simulink model "KD_cl_harness_forthao_breach"  (R2015a)
settings: Solver=ode45  StartTime=0  StopTime=50  FixedStep=0.01  MaxStep=0.005  RelTol=1e-4  AbsTol=1e-4
InitFcn:
  | load KD_const_coeffs_0624
  | load pexhat_stuff
  | load expcon
  | load thr_ff_map
undefined symbols (not defined in the file): c_0, c_1, c_100, c_1000, c_10000, c_1000inv, c_100inv, c_1_int, c_1d2p4, c_1p7, c_4400inv, c_5500inv, c_80, c_90, c_cal_phi, c_compmap, c_ctok, c_fflow_max, c_fflow_min, c_filt, c_flowdiv, c_flowmin, c_flowmult, c_inf, c_km1d2k, c_mm3tokgpers, c_n1, c_p00001, c_p01, c_p016, c_p1429, c_p1e9, c_p4167, c_p4d1p4, c_p5401, c_p9, c_pincomp, c_ra, c_rair, c_Rby1000, c_roacorr, c_rpmtoradpers, c_svrthrottle1, c_svrthrottle2, c_svrthrottlearg, c_svrthrottlebeta, c_ta_max, c_ta_min, c_V, c_vnliftmax, c_vnliftmin, Coefs, const, const_exhat, eegr_map, egrr_delay_init, epim_map, eplufin_ff_map, expcon, invta ... (+17)
libraries: simulink x5
(part 5 of 5)

== system KD_cl_harness_forthao_breach/ctrl_rb_explicit_20131031_v2/While_Iterator_Subsystem/newton/update ==
  dwdp : Inport
  error : Inport  Port=2
  Data Store Read1 : DataStoreRead  DataStoreName=man_pex_eps
  Data Store Read11 : DataStoreRead  DataStoreName=man_pex_eps
  Data Store Read16 : DataStoreRead  DataStoreName=man_use_LM
  Product2 : Product  Inputs=**  RndMeth=Zero
  Product3 : Product  Inputs=/*  RndMeth=Zero
  Product8 : Product  Inputs=/**  RndMeth=Zero
  Relational Operator7 : RelationalOperator  Operator=>  OutDataTypeStr=boolean
      settings: AttributesFormatString=%<Operator>
  Saturation1 : Saturate  UpperLimit=c_inf  LowerLimit=c_p1e9
      settings: AttributesFormatString=%<LowerLimit>\n%<UpperLimit>
  Saturation3 : Saturate  UpperLimit=c_inf  LowerLimit=c_p1e9
      settings: AttributesFormatString=%<LowerLimit>\n%<UpperLimit>
  Sum1 : Sum  Inputs=|++
  Sum2 : Sum  Inputs=|++
  Switch7 : Switch  Criteria=u2 ~= 0
      settings: AttributesFormatString=%<Criteria>
  man_pex_eps : Gain
  man_pex_eps1 : Gain
  man_use_LM : Gain
  zero8 : Constant  Value=0  OutDataTypeStr=single  SampleTime=-1
      settings: AttributesFormatString=%<Value>\n%<SampleTime>
  delta : Outport
  wires:
  Data Store Read11/1 -> man_pex_eps/1
  Sum2/1 -> Saturation3/1
  Saturation3/1 -> Product8/1
  Product2/1 -> Sum2/2
  error/1 -> [e]
  dwdp/1 -> [dwdp]
  [dwdp] -> Product2/1, Product8/2, Product2/2
  [e] -> Product8/3
  Data Store Read1/1 -> man_pex_eps1/1
  Sum1/1 -> Saturation1/1
  Saturation1/1 -> Product3/1
  [dwdp] -> Sum1/2
  [e] -> Product3/2
  zero8/1 -> Relational Operator7/2
  Data Store Read16/1 -> man_use_LM/1
  Relational Operator7/1 -> Switch7/2
  Product3/1 -> Switch7/3
  Product8/1 -> Switch7/1
  Switch7/1 -> delta/1
  man_pex_eps/1 -> Sum2/1
  man_pex_eps1/1 -> Sum1/1
  man_use_LM/1 -> Relational Operator7/1

== system KD_cl_harness_forthao_breach/ctrl_rb_explicit_20131031_v2/expcon/find_region/find_region ==
  u : Inport
  IC : Inport  Port=2
  Constant : Constant  DisableCoverage=on  Value=c_0  OutDataTypeStr=Inherit: Inherit via back propagation  PreserveConstantTs=on
      settings: AttributesFormatString=%<Value>
  g_zero_continue : RelationalOperator  Operator=>  OutDataTypeStr=boolean  InputSameDT=on
  get_region_violation : Subsystem
  if_region_1 : SwitchCase
  leq_check : Subsystem
  reg_register : UnitDelay  InitialCondition=c_1_int  SampleTime=-1
      settings: AttributesFormatString=%<X0>
  reg_update_merge : Merge  Inputs=3  InitialOutput=c_1_int
      settings: AttributesFormatString=%<InitialOutput>
  region_1feedthrough : Subsystem  TreatAsAtomicUnit=on
  region_iter : WhileIterator  MaxIters=expcon.Nr  ShowIterationPort=on
  rv_register : UnitDelay  InitialCondition=c_10000  SampleTime=-1
      settings: AttributesFormatString=%<X0>
  rv_update_merge : Merge  Inputs=3  InitialOutput=c_10000
      settings: AttributesFormatString=%<InitialOutput>
  region : Outport  InitialOutput=c_1_int
      settings: AttributesFormatString=%<InitialOutput>
  rv : Outport  Port=2  InitialOutput=c_10000
      settings: AttributesFormatString=%<InitialOutput>
  wires:
  region_iter/1 -> [iter]
  [iter] -> if_region_1/1, get_region_violation/1(region), leq_check/2(region_ind)
  IC/1 -> region_iter/2
  Constant/1 -> g_zero_continue/2
  [reg] -> reg_update_merge/1
  region_1feedthrough/2(region) -> [reg]
  [def] -> leq_check/Action
  if_region_1/2 -> [def]
  [u] -> get_region_violation/2(u)
  u/1 -> [u]
  get_region_violation/1(region_violation) -> region_1feedthrough/1(rvin), leq_check/1(rv_new)
  leq_check/1(rv_update_new) -> rv_update_merge/2
  rv_register/1 -> leq_check/3(rv_old)
  g_zero_continue/1 -> region_iter/1
  leq_check/3(region_update_new) -> reg_update_merge/2
  reg_register/1 -> leq_check/4(region_old)
  reg_update_merge/1 -> reg_register/1, region/1
  rv_update_merge/1 -> g_zero_continue/1, rv_register/1, rv/1
  region_1feedthrough/1(rvout) -> rv_update_merge/1
  if_region_1/1 -> region_1feedthrough/Action
  leq_check/2(rv_update_old) -> rv_update_merge/3
  leq_check/4(region_updateold) -> reg_update_merge/3

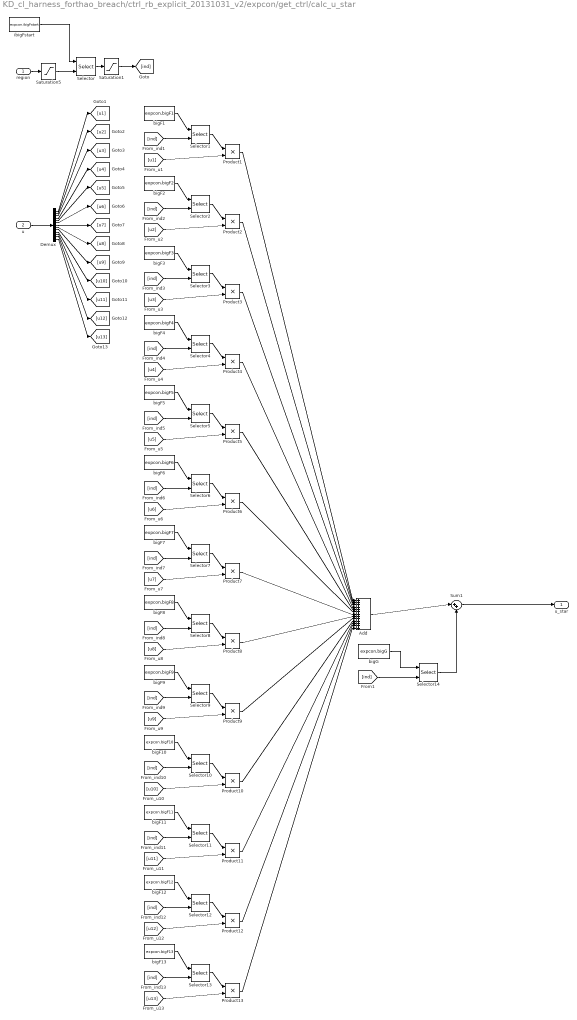
== system KD_cl_harness_forthao_breach/ctrl_rb_explicit_20131031_v2/expcon/get_ctrl/calc_u_star ==
  region : Inport
  u : Inport  Port=2
  Add : Sum  Inputs=+++++++++++++
  Demux : Demux  Outputs=13
  Product{1..13} (13 alike) : Product  RndMeth=Zero
  Saturation1 : Saturate  UpperLimit=307  LowerLimit=1
      settings: AttributesFormatString=%<LowerLimit>\n%<UpperLimit>
  Saturation5 : Saturate  UpperLimit=103  LowerLimit=1
      settings: AttributesFormatString=%<LowerLimit>\n%<UpperLimit>
  Selector : Selector  InputPortWidth=expcon.Nr  IndexOptions=Index vector (port)  Indices=[1 3]
  Selector{1..14} (14 alike) : Selector  InputPortWidth=309  IndexOptions=Starting index (port)  Indices=[1 3]  OutputSizes=3
  Sum1 : Sum  Inputs=|++
  bigF1 : Constant  Value=expcon.bigF1  OutDataTypeStr=single
      settings: AttributesFormatString=%<Value>
  bigF10 : Constant  Value=expcon.bigF10  OutDataTypeStr=single
      settings: AttributesFormatString=%<Value>
  bigF11 : Constant  Value=expcon.bigF11  OutDataTypeStr=single
      settings: AttributesFormatString=%<Value>
  bigF12 : Constant  Value=expcon.bigF12  OutDataTypeStr=single
      settings: AttributesFormatString=%<Value>
  bigF13 : Constant  Value=expcon.bigF13  OutDataTypeStr=single
      settings: AttributesFormatString=%<Value>
  bigF2 : Constant  Value=expcon.bigF2  OutDataTypeStr=single
      settings: AttributesFormatString=%<Value>
  bigF3 : Constant  Value=expcon.bigF3  OutDataTypeStr=single
      settings: AttributesFormatString=%<Value>
  bigF4 : Constant  Value=expcon.bigF4  OutDataTypeStr=single
      settings: AttributesFormatString=%<Value>
  bigF5 : Constant  Value=expcon.bigF5  OutDataTypeStr=single
      settings: AttributesFormatString=%<Value>
  bigF6 : Constant  Value=expcon.bigF6  OutDataTypeStr=single
      settings: AttributesFormatString=%<Value>
  bigF7 : Constant  Value=expcon.bigF7  OutDataTypeStr=single
      settings: AttributesFormatString=%<Value>
  bigF8 : Constant  Value=expcon.bigF8  OutDataTypeStr=single
      settings: AttributesFormatString=%<Value>
  bigF9 : Constant  Value=expcon.bigF9  OutDataTypeStr=single
      settings: AttributesFormatString=%<Value>
  bigG : Constant  Value=expcon.bigG  OutDataTypeStr=single
      settings: AttributesFormatString=%<Value>
  ibigFstart : Constant  Value=expcon.ibigFstart  OutDataTypeStr=single
      settings: AttributesFormatString=%<Value>
  u_star : Outport
  wires:
  Product13/1 -> Add/13
  [u13] -> Product13/2
  Selector13/1 -> Product13/1
  [ind] -> Selector13/2
  bigF13/1 -> Selector13/1
  Demux/13 -> [u13]
  Product12/1 -> Add/12
  [u12] -> Product12/2
  Selector12/1 -> Product12/1
  [ind] -> Selector12/2
  bigF12/1 -> Selector12/1
  Demux/12 -> [u12]
  Product11/1 -> Add/11
  [u11] -> Product11/2
  Selector11/1 -> Product11/1
  [ind] -> Selector11/2
  bigF11/1 -> Selector11/1
  Demux/11 -> [u11]
  Product10/1 -> Add/10
  [u10] -> Product10/2
  Selector10/1 -> Product10/1
  [ind] -> Selector10/2
  bigF10/1 -> Selector10/1
  Demux/10 -> [u10]
  Product9/1 -> Add/9
  [u9] -> Product9/2
  Selector9/1 -> Product9/1
  [ind] -> Selector9/2
  bigF9/1 -> Selector9/1
  Demux/9 -> [u9]
  Product8/1 -> Add/8
  [u8] -> Product8/2
  Selector8/1 -> Product8/1
  [ind] -> Selector8/2
  bigF8/1 -> Selector8/1
  Demux/8 -> [u8]
  Product7/1 -> Add/7
  [u7] -> Product7/2
  Selector7/1 -> Product7/1
  [ind] -> Selector7/2
  bigF7/1 -> Selector7/1
  Demux/7 -> [u7]
  Product6/1 -> Add/6
  [u6] -> Product6/2
  Selector6/1 -> Product6/1
  [ind] -> Selector6/2
  bigF6/1 -> Selector6/1
  Demux/6 -> [u6]
  Product5/1 -> Add/5
  [u5] -> Product5/2
  Selector5/1 -> Product5/1
  [ind] -> Selector5/2
  bigF5/1 -> Selector5/1
  Demux/5 -> [u5]
  Product4/1 -> Add/4
  [u4] -> Product4/2
  Selector4/1 -> Product4/1
  [ind] -> Selector4/2
  bigF4/1 -> Selector4/1
  Demux/4 -> [u4]
  Product3/1 -> Add/3
  [u3] -> Product3/2
  Selector3/1 -> Product3/1
  [ind] -> Selector3/2
  bigF3/1 -> Selector3/1
  Demux/3 -> [u3]
  Product2/1 -> Add/2
  [u2] -> Product2/2
  Selector2/1 -> Product2/1
  [ind] -> Selector2/2
  bigF2/1 -> Selector2/1
  Demux/2 -> [u2]
  Product1/1 -> Add/1
  [u1] -> Product1/2
  Selector1/1 -> Product1/1
  [ind] -> Selector1/2
  bigF1/1 -> Selector1/1
  Demux/1 -> [u1]
  Saturation1/1 -> [ind]
  Saturation5/1 -> Selector/2
  Add/1 -> Sum1/1
  [ind] -> Selector14/2
  u/1 -> Demux/1
  Selector14/1 -> Sum1/2
  bigG/1 -> Selector14/1
  Sum1/1 -> u_star/1
  Selector/1 -> Saturation1/1
  ibigFstart/1 -> Selector/1
  region/1 -> Saturation5/1

== system KD_cl_harness_forthao_breach/ctrl_rb_explicit_20131031_v2/invert_flow/valve_inversion/Cal_phi1 ==
  Pa : Inport
  Ro_a : Inport  Port=2
  Abs : Abs
  Gain1 : Gain  Gain=c_cal_phi  SaturateOnIntegerOverflow=on  OutDataTypeStr=Inherit: Same as input  ParamDataTypeStr=Inherit: Same as input
  Product4 : Product  Inputs=**  SaturateOnIntegerOverflow=on  RndMeth=Zero  InputSameDT=on  OutDataTypeStr=Inherit: Same as first input
  Sqrt : Sqrt  AlgorithmType=Newton-Raphson  SaturateOnIntegerOverflow=on
  phi : Outport
  wires:
  Abs/1 -> Sqrt/1
  Gain1/1 -> Abs/1
  Sqrt/1 -> phi/1
  Ro_a/1 -> Product4/2
  Pa/1 -> Product4/1
  Product4/1 -> Gain1/1

== system KD_cl_harness_forthao_breach/ctrl_rb_explicit_20131031_v2/ntestimator/Throttle_Model/Air_Model_map_use ==
  TA_deg : Inport
  Ne_rpm : Inport  Port=2
  Pim_Pa : Inport  Port=3
  Ta_K : Inport  Port=4
  R_a : Inport  Port=5
  wegrthr : Inport  Port=6
  Forward_Flow : Subsystem
  Product1 : Product  Inputs=*//  SaturateOnIntegerOverflow=on  RndMeth=Zero  InputSameDT=on  OutDataTypeStr=Inherit: Same as first input
  Saturation1 : Saturate  UpperLimit=c_inf  LowerLimit=c_p1e9
      settings: AttributesFormatString=%<LowerLimit>\n%<UpperLimit>
  Saturation5 : Saturate  UpperLimit=c_inf  LowerLimit=c_p1e9
      settings: AttributesFormatString=%<LowerLimit>\n%<UpperLimit>
  one : Constant  OutDataTypeStr=single  SampleTime=sample_time
      settings: AttributesFormatString=%<Value>\n%<SampleTime>
  p_pre_throttle : Outport
  wires:
  Product1/1 -> Forward_Flow/1(Ro_a)
  TA_deg/1 -> Forward_Flow/2(TA_deg)
  Pim_Pa/1 -> Forward_Flow/4(Pm)
  Ta_K/1 -> Saturation5/1
  R_a/1 -> Saturation1/1
  one/1 -> Product1/1
  Ne_rpm/1 -> Forward_Flow/3(Ne_rpm)
  wegrthr/1 -> Forward_Flow/5(wegrthr)
  Forward_Flow/1(p_pre_throttle) -> p_pre_throttle/1
  Saturation5/1 -> Product1/2
  Saturation1/1 -> Product1/3

== system KD_cl_harness_forthao_breach/ctrl_rb_explicit_20131031_v2/set_point_maps/intake_pressure_map/boost_pressure_map ==
  fuel_rate_mm3perst : Inport
  engine_speed : Inport  Port=2
  epimbs_map : Lookup2D  RowIndex=epim_map.x  ColumnIndex=epim_map.y  Table=epim_map.z  LookUpMeth=Interpolation-Use End Values
      settings: AttributesFormatString=%<LookUpMeth>\n%<RowIndex>\n%<ColumnIndex>
  intake_manifold_pressure : Outport
  wires:
  epimbs_map/1 -> intake_manifold_pressure/1
  fuel_rate_mm3perst/1 -> epimbs_map/2
  engine_speed/1 -> epimbs_map/1

== system KD_cl_harness_forthao_breach/EGR Throttle/EGR Throttle/Throttle Model2/Air Model_map_use/Back-Flow ==
  TA[deg] : Inport
  Ne[rpm] : Inport  Port=2
  Ro_m : Inport  Port=3
  Pa : Inport  Port=4
  Pm : Inport  Port=5
  Cal phi1 : Subsystem
  Constant1 : Constant  Value=(const.k/(2*(const.k+1)))^0.5
  Constant2 : Constant  Value=SVR_throttle.Beta
  Constant6 : Constant  Value=SVR_throttle.num_SV
  Constant7 : Constant  Value=SVR_throttle.SV
  Constant8 : Constant  Value=SVR_throttle.arg
  Gain : Gain  Gain=1/100
  Gain1 : Gain  Gain=1/5500
  Mux : Mux  Inputs=2
  Phi1 : Fcn  Expr=sqrt(((const.k-1)/(2*const.k)*(1-u)+u)*(1-u))
  Pm/Pa1 : Product  Inputs=/*  SaturateOnIntegerOverflow=on  RndMeth=Zero  InputSameDT=on  OutDataTypeStr=Inherit: Same as first input
  SVR_throttle : MATLAB Function  TreatAsAtomicUnit=on
  Saturation : Saturate  UpperLimit=inf  LowerLimit=0
  Saturation1 : Saturate  UpperLimit=1.0  LowerLimit=1/(const.k+1)
  Switch1 : Switch  Criteria=u2 > Threshold  Threshold=1/(const.k+1)
  correct flow2 : Product  Inputs=***  SaturateOnIntegerOverflow=on  RndMeth=Zero  InputSameDT=on  OutDataTypeStr=Inherit: Same as first input
  tokgps1 : Gain  Gain=1/1000
  mt_dot[kg/s] : Outport
  wires:
  Cal phi1/1(phi) -> correct flow2/1
  Constant1/1 -> Switch1/3
  Switch1/1 -> correct flow2/3
  Saturation1/1 -> Phi1/1
  Phi1/1 -> Switch1/1
  correct flow2/1 -> tokgps1/1
  tokgps1/1 -> mt_dot[kg/s]/1
  Pm/Pa1/1 -> Switch1/2, Saturation1/1
  Pm/1 -> Pm/Pa1/1, Cal phi1/1(Pm)
  Pa/1 -> Pm/Pa1/2
  Ro_m/1 -> Cal phi1/2(Ro_m)
  SVR_throttle/1(B_A_spd) -> Saturation/1
  TA[deg]/1 -> Gain/1
  Gain/1 -> Mux/1
  Gain1/1 -> Mux/2
  Ne[rpm]/1 -> Gain1/1
  Constant6/1 -> SVR_throttle/2(num_SV)
  Constant2/1 -> SVR_throttle/3(Beta)
  Constant7/1 -> SVR_throttle/4(SV)
  Constant8/1 -> SVR_throttle/5(arg)
  Mux/1 -> SVR_throttle/1(u)
  Saturation/1 -> correct flow2/2

== system KD_cl_harness_forthao_breach/EGR Throttle/EGR Throttle/Throttle Model2/Air Model_map_use/Forward-Flow ==
  Ro_a : Inport
  TA[deg] : Inport  Port=2
  Ne[rpm] : Inport  Port=3
  Pa : Inport  Port=4
  Pm : Inport  Port=5
  Cal phi : Subsystem
  Constant1 : Constant  Value=(const.k/(2*(const.k+1)))^0.5
  Constant2 : Constant  Value=SVR_throttle.Beta
  Constant6 : Constant  Value=SVR_throttle.num_SV
  Constant7 : Constant  Value=SVR_throttle.SV
  Constant8 : Constant  Value=SVR_throttle.arg
  Gain : Gain  Gain=1/100
  Gain1 : Gain  Gain=1/5500
  Mux : Mux  Inputs=2
  Phi1 : Fcn  Expr=sqrt(((const.k-1)/(2*const.k)*(1-u)+u)*(1-u))
  Pm/Pa1 : Product  Inputs=*/  SaturateOnIntegerOverflow=on  RndMeth=Zero  InputSameDT=on  OutDataTypeStr=Inherit: Same as first input
  SVR_throttle : MATLAB Function  TreatAsAtomicUnit=on
  Saturation : Saturate  UpperLimit=inf  LowerLimit=0
  Saturation1 : Saturate  UpperLimit=1.0  LowerLimit=1/(const.k+1)
  Switch1 : Switch  Criteria=u2 > Threshold  Threshold=1/(const.k+1)
  correct flow2 : Product  Inputs=***  SaturateOnIntegerOverflow=on  RndMeth=Zero  InputSameDT=on  OutDataTypeStr=Inherit: Same as first input
  tokgps1 : Gain  Gain=1/1000
  mt_dot[kg/s] : Outport
  wires:
  Cal phi/1(phi) -> correct flow2/1
  Constant1/1 -> Switch1/3
  Switch1/1 -> correct flow2/3
  Saturation1/1 -> Phi1/1
  Phi1/1 -> Switch1/1
  correct flow2/1 -> tokgps1/1
  tokgps1/1 -> mt_dot[kg/s]/1
  Pm/Pa1/1 -> Switch1/2, Saturation1/1
  Pm/1 -> Pm/Pa1/1
  Pa/1 -> Pm/Pa1/2, Cal phi/1(Pa)
  Ro_a/1 -> Cal phi/2(Ro_a)
  Mux/1 -> SVR_throttle/1(u)
  TA[deg]/1 -> Gain/1
  Gain/1 -> Mux/1
  Gain1/1 -> Mux/2
  Ne[rpm]/1 -> Gain1/1
  SVR_throttle/1(B_A_spd) -> Saturation/1
  Constant6/1 -> SVR_throttle/2(num_SV)
  Constant2/1 -> SVR_throttle/3(Beta)
  Constant7/1 -> SVR_throttle/4(SV)
  Constant8/1 -> SVR_throttle/5(arg)
  Saturation/1 -> correct flow2/2  "B(TA)(g/s)"

== system KD_cl_harness_forthao_breach/EGR Valve/SVR EGR/EGR_model/Air Model_map_use/Back-Flow ==
  TA[deg] : Inport
  Ne[rpm] : Inport  Port=2
  Ro_m : Inport  Port=3
  Pa : Inport  Port=4
  Pm : Inport  Port=5
  Cal phi1 : Subsystem
  Constant1 : Constant  Value=(const.k/(2*(const.k+1)))^0.5
  Constant2 : Constant  Value=SVR_EGR.Beta
  Constant6 : Constant  Value=SVR_EGR.num_SV
  Constant7 : Constant  Value=SVR_EGR.SV
  Constant8 : Constant  Value=SVR_EGR.arg
  Gain : Gain  Gain=1/100
  Gain1 : Gain  Gain=1/5500
  Gain2 : Gain  Gain=1/1000
  Mux : Mux  Inputs=2
  Phi1 : Fcn  Expr=sqrt(((const.k-1)/(2*const.k)*(1-u)+u)*(1-u))
  Pm/Pa1 : Product  Inputs=/*  SaturateOnIntegerOverflow=on  RndMeth=Zero  InputSameDT=on  OutDataTypeStr=Inherit: Same as first input
  SVR_EGR : MATLAB Function  TreatAsAtomicUnit=on
  Saturation : Saturate  UpperLimit=inf  LowerLimit=0
  Saturation1 : Saturate  UpperLimit=1.0  LowerLimit=1/(const.k+1)
  Switch1 : Switch  Criteria=u2 > Threshold  Threshold=1/(const.k+1)
  correct flow2 : Product  Inputs=***  SaturateOnIntegerOverflow=on  RndMeth=Zero  InputSameDT=on  OutDataTypeStr=Inherit: Same as first input
  mt_dot[kg/s] : Outport
  wires:
  Gain2/1 -> mt_dot[kg/s]/1
  Mux/1 -> SVR_EGR/1(u)
  Constant8/1 -> SVR_EGR/5(arg)
  Constant7/1 -> SVR_EGR/4(SV)
  Constant2/1 -> SVR_EGR/3(Beta)
  Constant6/1 -> SVR_EGR/2(num_SV)
  Ne[rpm]/1 -> Gain1/1
  Gain1/1 -> Mux/2
  Gain/1 -> Mux/1
  TA[deg]/1 -> Gain/1
  SVR_EGR/1(B_A_spd) -> Saturation/1
  Ro_m/1 -> Cal phi1/2(Ro_m)
  Pa/1 -> Pm/Pa1/2
  Pm/1 -> Cal phi1/1(Pm), Pm/Pa1/1
  Pm/Pa1/1 -> Saturation1/1, Switch1/2
  correct flow2/1 -> Gain2/1
  Phi1/1 -> Switch1/1
  Saturation1/1 -> Phi1/1
  Switch1/1 -> correct flow2/3
  Constant1/1 -> Switch1/3
  Cal phi1/1(phi) -> correct flow2/1
  Saturation/1 -> correct flow2/2

== system KD_cl_harness_forthao_breach/EGR Valve/SVR EGR/EGR_model/Air Model_map_use/Forward-Flow ==
  Ro_a : Inport
  TA[deg] : Inport  Port=2
  Ne[rpm] : Inport  Port=3
  Pa : Inport  Port=4
  Pm : Inport  Port=5
  Cal phi : Subsystem
  Constant1 : Constant  Value=(const.k/(2*(const.k+1)))^0.5
  Constant3 : Constant  Value=SVR_EGR.Beta
  Constant4 : Constant  Value=SVR_EGR.num_SV
  Constant5 : Constant  Value=SVR_EGR.SV
  Constant9 : Constant  Value=SVR_EGR.arg
  Gain : Gain  Gain=1/100
  Gain1 : Gain  Gain=1/4400
  Gain2 : Gain  Gain=1/1000
  Mux : Mux  Inputs=2
  Phi1 : Fcn  Expr=sqrt(((const.k-1)/(2*const.k)*(1-u)+u)*(1-u))
  Pm/Pa1 : Product  Inputs=*/  SaturateOnIntegerOverflow=on  RndMeth=Zero  InputSameDT=on  OutDataTypeStr=Inherit: Same as first input
  SVR_EGR : MATLAB Function  TreatAsAtomicUnit=on
  Saturation : Saturate  UpperLimit=inf  LowerLimit=0
  Saturation1 : Saturate  UpperLimit=1.0  LowerLimit=1/(const.k+1)
  Switch1 : Switch  Criteria=u2 > Threshold  Threshold=1/(const.k+1)
  correct flow2 : Product  Inputs=***  SaturateOnIntegerOverflow=on  RndMeth=Zero  InputSameDT=on  OutDataTypeStr=Inherit: Same as first input
  mt_dot[kg/s] : Outport
  wires:
  Gain2/1 -> mt_dot[kg/s]/1
  Constant9/1 -> SVR_EGR/5(arg)
  Constant5/1 -> SVR_EGR/4(SV)
  Constant3/1 -> SVR_EGR/3(Beta)
  Constant4/1 -> SVR_EGR/2(num_SV)
  SVR_EGR/1(B_A_spd) -> Saturation/1
  Ne[rpm]/1 -> Gain1/1
  Gain1/1 -> Mux/2
  Gain/1 -> Mux/1
  TA[deg]/1 -> Gain/1
  Mux/1 -> SVR_EGR/1(u)
  Ro_a/1 -> Cal phi/2(Ro_a)
  Pa/1 -> Cal phi/1(Pa), Pm/Pa1/2
  Pm/1 -> Pm/Pa1/1
  Pm/Pa1/1 -> Saturation1/1, Switch1/2
  correct flow2/1 -> Gain2/1
  Phi1/1 -> Switch1/1
  Saturation1/1 -> Phi1/1
  Switch1/1 -> correct flow2/3
  Constant1/1 -> Switch1/3
  Cal phi/1(phi) -> correct flow2/1
  Saturation/1 -> correct flow2/2  "B(TA)(g/s)"

== system KD_cl_harness_forthao_breach/ctrl_rb_explicit_20131031_v2/EGR_max_flow/Air_Model_map_use/Forward_Flow/Cal_phi ==
  Pa : Inport
  Ro_a : Inport  Port=2
  Abs : Abs
  Gain2 : Gain  Gain=c_cal_phi  ParamDataTypeStr=single  SaturateOnIntegerOverflow=on  OutDataTypeStr=Inherit: Same as input
  Product4 : Product  Inputs=**  OutDataTypeStr=single  SaturateOnIntegerOverflow=on  RndMeth=Zero  InputSameDT=on
  Sqrt : Sqrt  AlgorithmType=Newton-Raphson  SaturateOnIntegerOverflow=on
  phi : Outport
  wires:
  Sqrt/1 -> phi/1
  Abs/1 -> Sqrt/1
  Product4/1 -> Gain2/1
  Gain2/1 -> Abs/1
  Pa/1 -> Product4/1
  Ro_a/1 -> Product4/2

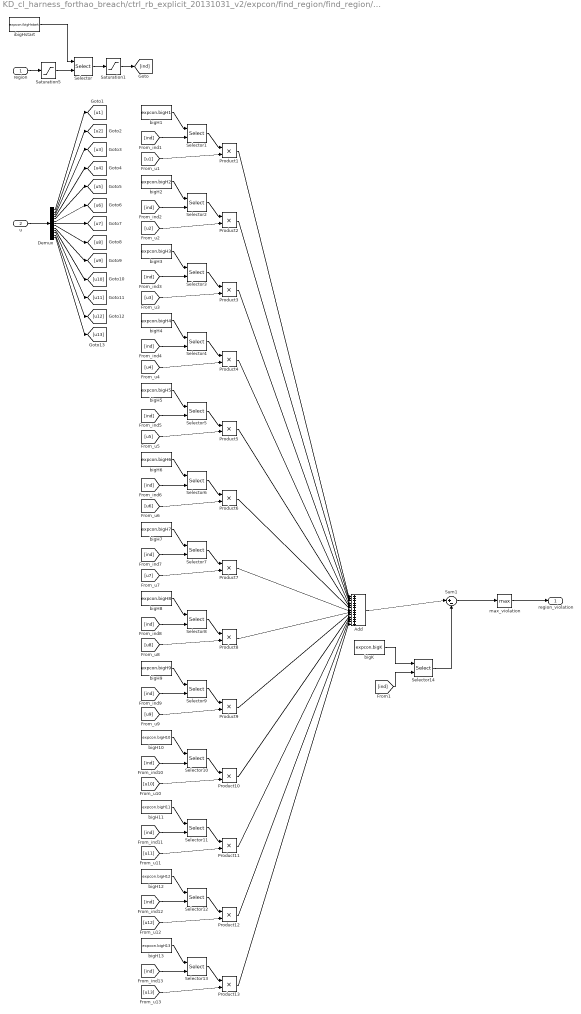
== system KD_cl_harness_forthao_breach/ctrl_rb_explicit_20131031_v2/expcon/find_region/find_region/get_region_violation ==
  region : Inport
  u : Inport  Port=2
  Add : Sum  Inputs=+++++++++++++
  Demux : Demux  Outputs=13
  Product{1..13} (13 alike) : Product  RndMeth=Zero
  Saturation1 : Saturate  UpperLimit=1021  LowerLimit=1
      settings: AttributesFormatString=%<LowerLimit>\n%<UpperLimit>
  Saturation5 : Saturate  UpperLimit=103  LowerLimit=1
      settings: AttributesFormatString=%<LowerLimit>\n%<UpperLimit>
  Selector : Selector  InputPortWidth=expcon.Nr  IndexOptions=Index vector (port)  Indices=[1 3]
  Selector{1..14} (14 alike) : Selector  InputPortWidth=1030  IndexOptions=Starting index (port)  Indices=[1 3]  OutputSizes=10
  Sum1 : Sum  Inputs=|+-
  bigH1 : Constant  Value=expcon.bigH1  OutDataTypeStr=single
      settings: AttributesFormatString=%<Value>
  bigH10 : Constant  Value=expcon.bigH10  OutDataTypeStr=single
      settings: AttributesFormatString=%<Value>
  bigH11 : Constant  Value=expcon.bigH11  OutDataTypeStr=single
      settings: AttributesFormatString=%<Value>
  bigH12 : Constant  Value=expcon.bigH12  OutDataTypeStr=single
      settings: AttributesFormatString=%<Value>
  bigH13 : Constant  Value=expcon.bigH13  OutDataTypeStr=single
      settings: AttributesFormatString=%<Value>
  bigH2 : Constant  Value=expcon.bigH2  OutDataTypeStr=single
      settings: AttributesFormatString=%<Value>
  bigH3 : Constant  Value=expcon.bigH3  OutDataTypeStr=single
      settings: AttributesFormatString=%<Value>
  bigH4 : Constant  Value=expcon.bigH4  OutDataTypeStr=single
      settings: AttributesFormatString=%<Value>
  bigH5 : Constant  Value=expcon.bigH5  OutDataTypeStr=single
      settings: AttributesFormatString=%<Value>
  bigH6 : Constant  Value=expcon.bigH6  OutDataTypeStr=single
      settings: AttributesFormatString=%<Value>
  bigH7 : Constant  Value=expcon.bigH7  OutDataTypeStr=single
      settings: AttributesFormatString=%<Value>
  bigH8 : Constant  Value=expcon.bigH8  OutDataTypeStr=single
      settings: AttributesFormatString=%<Value>
  bigH9 : Constant  Value=expcon.bigH9  OutDataTypeStr=single
      settings: AttributesFormatString=%<Value>
  bigK : Constant  Value=expcon.bigK  OutDataTypeStr=single
      settings: AttributesFormatString=%<Value>
  ibigHstart : Constant  Value=expcon.ibigHstart  OutDataTypeStr=single
      settings: AttributesFormatString=%<Value>
  max_violation : MinMax  Function=max
      settings: AttributesFormatString=%<Function>
  region_violation : Outport
  wires:
  Product13/1 -> Add/13
  [u13] -> Product13/2
  Selector13/1 -> Product13/1
  [ind] -> Selector13/2
  bigH13/1 -> Selector13/1
  Demux/13 -> [u13]
  Product12/1 -> Add/12
  [u12] -> Product12/2
  Selector12/1 -> Product12/1
  [ind] -> Selector12/2
  bigH12/1 -> Selector12/1
  Demux/12 -> [u12]
  Product11/1 -> Add/11
  [u11] -> Product11/2
  Selector11/1 -> Product11/1
  [ind] -> Selector11/2
  bigH11/1 -> Selector11/1
  Demux/11 -> [u11]
  Product10/1 -> Add/10
  [u10] -> Product10/2
  Selector10/1 -> Product10/1
  [ind] -> Selector10/2
  bigH10/1 -> Selector10/1
  Demux/10 -> [u10]
  Product9/1 -> Add/9
  [u9] -> Product9/2
  Selector9/1 -> Product9/1
  [ind] -> Selector9/2
  bigH9/1 -> Selector9/1
  Demux/9 -> [u9]
  Product8/1 -> Add/8
  [u8] -> Product8/2
  Selector8/1 -> Product8/1
  [ind] -> Selector8/2
  bigH8/1 -> Selector8/1
  Demux/8 -> [u8]
  Product7/1 -> Add/7
  [u7] -> Product7/2
  Selector7/1 -> Product7/1
  [ind] -> Selector7/2
  bigH7/1 -> Selector7/1
  Demux/7 -> [u7]
  Product6/1 -> Add/6
  [u6] -> Product6/2
  Selector6/1 -> Product6/1
  [ind] -> Selector6/2
  bigH6/1 -> Selector6/1
  Demux/6 -> [u6]
  Product5/1 -> Add/5
  [u5] -> Product5/2
  Selector5/1 -> Product5/1
  [ind] -> Selector5/2
  bigH5/1 -> Selector5/1
  Demux/5 -> [u5]
  Product4/1 -> Add/4
  [u4] -> Product4/2
  Selector4/1 -> Product4/1
  [ind] -> Selector4/2
  bigH4/1 -> Selector4/1
  Demux/4 -> [u4]
  Product3/1 -> Add/3
  [u3] -> Product3/2
  Selector3/1 -> Product3/1
  [ind] -> Selector3/2
  bigH3/1 -> Selector3/1
  Demux/3 -> [u3]
  Product2/1 -> Add/2
  [u2] -> Product2/2
  Selector2/1 -> Product2/1
  [ind] -> Selector2/2
  bigH2/1 -> Selector2/1
  Demux/2 -> [u2]
  Product1/1 -> Add/1
  [u1] -> Product1/2
  Selector1/1 -> Product1/1
  [ind] -> Selector1/2
  bigH1/1 -> Selector1/1
  Demux/1 -> [u1]
  Saturation1/1 -> [ind]
  Saturation5/1 -> Selector/2
  Add/1 -> Sum1/1
  [ind] -> Selector14/2
  u/1 -> Demux/1
  Selector14/1 -> Sum1/2
  bigK/1 -> Selector14/1
  max_violation/1 -> region_violation/1
  Sum1/1 -> max_violation/1
  Selector/1 -> Saturation1/1
  ibigHstart/1 -> Selector/1
  region/1 -> Saturation5/1

== system KD_cl_harness_forthao_breach/ctrl_rb_explicit_20131031_v2/expcon/find_region/find_region/leq_check ==
  rv_new : Inport
  region_ind : Inport  Port=2
  rv_old : Inport  Port=3
  region_old : Inport  Port=4
  Action Port : ActionPort  ActionType=default
  if_new_min_rv : If  NumInputs=2  IfExpression=u1 < u2
  new_region : Subsystem  TreatAsAtomicUnit=on
  old_region : Subsystem  TreatAsAtomicUnit=on
  rv_update_new : Outport
  rv_update_old : Outport  Port=2
  region_update_new : Outport  Port=3
  region_updateold : Outport  Port=4
  wires:
  if_new_min_rv/2 -> [els]
  [els] -> old_region/Action
  [rv] -> if_new_min_rv/2
  rv_old/1 -> old_region/1(rv_in), [rv]
  rv_new/1 -> if_new_min_rv/1, new_region/1(rv_in)
  if_new_min_rv/1 -> new_region/Action
  region_ind/1 -> new_region/2(region_in)
  new_region/1(rv_out) -> rv_update_new/1
  region_old/1 -> old_region/2(region_in)
  new_region/2(region_out) -> region_update_new/1
  old_region/1(rv_out) -> rv_update_old/1
  old_region/2(region_out) -> region_updateold/1

== system KD_cl_harness_forthao_breach/ctrl_rb_explicit_20131031_v2/expcon/find_region/find_region/region_1feedthrough ==
  rvin : Inport
  Action Port : ActionPort  ActionType=case
  region_1 : Constant  Value=c_1_int  OutDataTypeStr=int32
  rvout : Outport
  region : Outport  Port=2  InitialOutput=1
      settings: AttributesFormatString=%<InitialOutput>
  wires:
  rvin/1 -> rvout/1
  region_1/1 -> region/1

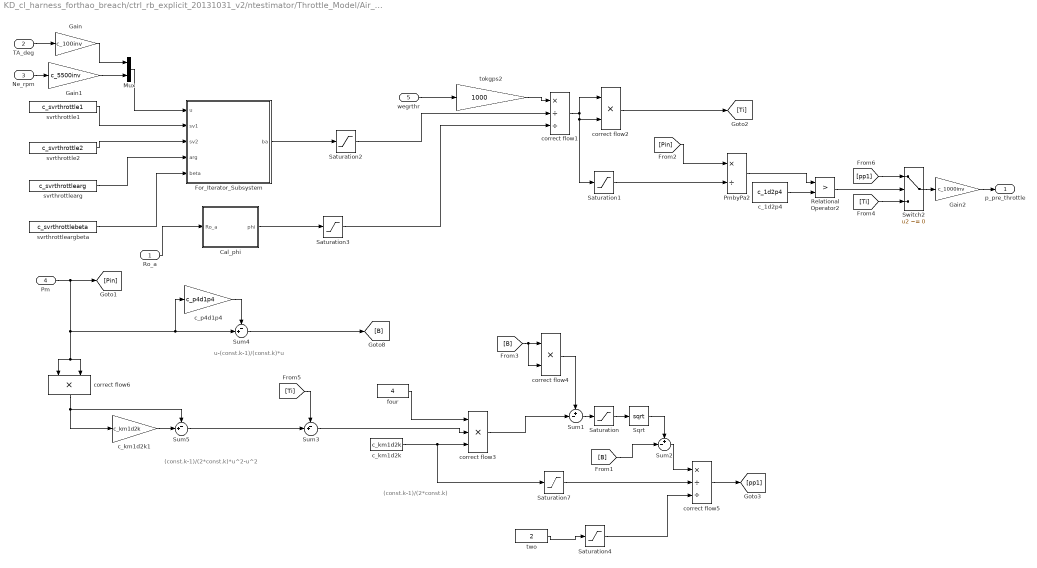
== system KD_cl_harness_forthao_breach/ctrl_rb_explicit_20131031_v2/ntestimator/Throttle_Model/Air_Model_map_use/Forward_Flow ==
  note: u-(const.k-1)/(const.k)*u
  note: (const.k-1)/(2*const.k)*u^2-u^2
  note: (const.k-1)/(2*const.k)
  Ro_a : Inport
  TA_deg : Inport  Port=2
  Ne_rpm : Inport  Port=3
  Pm : Inport  Port=4
  wegrthr : Inport  Port=5
  Cal_phi : Subsystem
  For_Iterator_Subsystem : Subsystem  TreatAsAtomicUnit=on
  Gain : Gain  Gain=c_100inv
      settings: AttributesFormatString=%<Gain>
  Gain1 : Gain  Gain=c_5500inv
      settings: AttributesFormatString=%<Gain>
  Gain2 : Gain  Gain=c_1000inv
      settings: AttributesFormatString=%<Gain>
  Mux : Mux  Inputs=2
  PmbyPa2 : Product  Inputs=*/  SaturateOnIntegerOverflow=on  RndMeth=Zero  InputSameDT=on  OutDataTypeStr=Inherit: Same as first input
  Relational Operator2 : RelationalOperator  Operator=>  OutDataTypeStr=boolean
      settings: AttributesFormatString=%<Operator>
  Saturation : Saturate  UpperLimit=c_inf  LowerLimit=0
      settings: AttributesFormatString=%<LowerLimit>\n%<UpperLimit>
  Saturation{1..4,7} (5 alike) : Saturate  UpperLimit=c_inf  LowerLimit=c_p1e9
      settings: AttributesFormatString=%<LowerLimit>\n%<UpperLimit>
  Sqrt : Sqrt  AlgorithmType=Newton-Raphson  SaturateOnIntegerOverflow=on
  Sum1 : Sum  Inputs=+-|
  Sum2 : Sum  Inputs=+-|
  Sum3 : Sum  Inputs=-+|
  Sum4 : Sum  Inputs=-+|
  Sum5 : Sum  Inputs=-+|
  Switch2 : Switch  Criteria=u2 ~= 0
      settings: AttributesFormatString=%<Criteria>
  c_1d2p4 : Constant  Value=c_1d2p4  OutDataTypeStr=single  SampleTime=sample_time
      settings: AttributesFormatString=%<Value>\n%<SampleTime>
  c_km1d2k : Constant  Value=c_km1d2k  OutDataTypeStr=single  SampleTime=sample_time
      settings: AttributesFormatString=%<Value>\n%<SampleTime>
  c_km1d2k1 : Gain  Gain=c_km1d2k
  c_p4d1p4 : Gain  Gain=c_p4d1p4
  correct flow1 : Product  Inputs=*//  SaturateOnIntegerOverflow=on  RndMeth=Zero  InputSameDT=on  OutDataTypeStr=Inherit: Same as first input
  correct flow2 : Product  Inputs=**  SaturateOnIntegerOverflow=on  RndMeth=Zero  InputSameDT=on  OutDataTypeStr=Inherit: Same as first input
  correct flow3 : Product  Inputs=***  SaturateOnIntegerOverflow=on  RndMeth=Zero  InputSameDT=on  OutDataTypeStr=Inherit: Same as first input
  correct flow4 : Product  Inputs=**  SaturateOnIntegerOverflow=on  RndMeth=Zero  InputSameDT=on  OutDataTypeStr=Inherit: Same as first input
  correct flow5 : Product  Inputs=*//  SaturateOnIntegerOverflow=on  RndMeth=Zero  InputSameDT=on  OutDataTypeStr=Inherit: Same as first input
  correct flow6 : Product  Inputs=**  SaturateOnIntegerOverflow=on  RndMeth=Zero  InputSameDT=on  OutDataTypeStr=Inherit: Same as first input
  four : Constant  Value=4  OutDataTypeStr=single  SampleTime=sample_time
      settings: AttributesFormatString=%<Value>\n%<SampleTime>
  svrthrottle1 : Constant  Value=c_svrthrottle1  OutDataTypeStr=single  SampleTime=sample_time
      settings: AttributesFormatString=%<Value>\n%<SampleTime>
  svrthrottle2 : Constant  Value=c_svrthrottle2  OutDataTypeStr=single  SampleTime=sample_time
      settings: AttributesFormatString=%<Value>\n%<SampleTime>
  svrthrottlearg : Constant  Value=c_svrthrottlearg  OutDataTypeStr=single  SampleTime=sample_time
      settings: AttributesFormatString=%<Value>\n%<SampleTime>
  svrthrottleargbeta : Constant  Value=c_svrthrottlebeta  OutDataTypeStr=single  SampleTime=sample_time
      settings: AttributesFormatString=%<Value>\n%<SampleTime>
  tokgps2 : Gain  Gain=1000
  two : Constant  Value=2  OutDataTypeStr=single  SampleTime=sample_time
      settings: AttributesFormatString=%<Value>\n%<SampleTime>
  p_pre_throttle : Outport  OutDataTypeStr=single
  wires:
  Cal_phi/1(phi) -> Saturation3/1
  Pm/1 -> Sum4/2, c_p4d1p4/1, correct flow6/1, correct flow6/2, [Pin]
  Ro_a/1 -> Cal_phi/1(Ro_a)
  Mux/1 -> For_Iterator_Subsystem/1(u)
  TA_deg/1 -> Gain/1
  Gain/1 -> Mux/1
  Gain1/1 -> Mux/2
  Ne_rpm/1 -> Gain1/1
  wegrthr/1 -> tokgps2/1
  tokgps2/1 -> correct flow1/1
  correct flow1/1 -> correct flow2/1, correct flow2/2, Saturation1/1
  four/1 -> correct flow3/1
  c_km1d2k/1 -> correct flow3/3, Saturation7/1
  correct flow3/1 -> Sum1/2
  Sum1/1 -> Saturation/1
  Sqrt/1 -> Sum2/1
  Sum2/1 -> correct flow5/1
  two/1 -> Saturation4/1
  Switch2/1 -> Gain2/1
  Gain2/1 -> p_pre_throttle/1
  correct flow4/1 -> Sum1/1
  Saturation1/1 -> PmbyPa2/2
  Saturation2/1 -> correct flow1/2
  Saturation3/1 -> correct flow1/3
  Saturation7/1 -> correct flow5/2
  Saturation4/1 -> correct flow5/3
  For_Iterator_Subsystem/1(ba) -> Saturation2/1
  Sum4/1 -> [B]
  [B] -> correct flow4/1, correct flow4/2
  [B] -> Sum2/2
  [Pin] -> PmbyPa2/1
  correct flow2/1 -> [Ti]
  [Ti] -> Switch2/3
  [Ti] -> Sum3/1
  correct flow5/1 -> [pp1]
  [pp1] -> Switch2/1
  Sum3/1 -> correct flow3/2
  Saturation/1 -> Sqrt/1
  svrthrottle1/1 -> For_Iterator_Subsystem/2(sv1)
  svrthrottle2/1 -> For_Iterator_Subsystem/3(sv2)
  svrthrottlearg/1 -> For_Iterator_Subsystem/4(arg)
  svrthrottleargbeta/1 -> For_Iterator_Subsystem/5(beta)
  Sum5/1 -> Sum3/2
  correct flow6/1 -> c_km1d2k1/1, Sum5/1
  c_1d2p4/1 -> Relational Operator2/2
  PmbyPa2/1 -> Relational Operator2/1
  Relational Operator2/1 -> Switch2/2
  c_p4d1p4/1 -> Sum4/1
  c_km1d2k1/1 -> Sum5/2

== system KD_cl_harness_forthao_breach/EGR Throttle/EGR Throttle/Throttle Model2/Air Model_map_use/Back-Flow/Cal phi1 ==
  Pm : Inport
  Ro_m : Inport  Port=2
  Gain2 : Gain  Gain=1/(const.Pcab*const.Pcab/const.Rair/const.Tcab)  SaturateOnIntegerOverflow=on  OutDataTypeStr=Inherit: Same as input  ParamDataTypeStr=Inherit: Same as input
  Math Function : Sqrt  Operator=signedSqrt  AlgorithmType=Newton-Raphson  SaturateOnIntegerOverflow=on
  Product4 : Product  Inputs=**  SaturateOnIntegerOverflow=on  RndMeth=Zero  InputSameDT=on  OutDataTypeStr=Inherit: Same as first input
  phi : Outport
  wires:
  Math Function/1 -> phi/1
  Ro_m/1 -> Product4/2
  Pm/1 -> Product4/1
  Gain2/1 -> Math Function/1
  Product4/1 -> Gain2/1

== system KD_cl_harness_forthao_breach/EGR Throttle/EGR Throttle/Throttle Model2/Air Model_map_use/Forward-Flow/Cal phi ==
  Pa : Inport
  Ro_a : Inport  Port=2
  Gain2 : Gain  Gain=1/(const.Pcab*const.Pcab/const.Rair/const.Tcab)  SaturateOnIntegerOverflow=on  OutDataTypeStr=Inherit: Same as input  ParamDataTypeStr=Inherit: Same as input
  Math Function : Sqrt  Operator=signedSqrt  AlgorithmType=Newton-Raphson  SaturateOnIntegerOverflow=on
  Product4 : Product  Inputs=**  SaturateOnIntegerOverflow=on  RndMeth=Zero  InputSameDT=on  OutDataTypeStr=Inherit: Same as first input
  phi : Outport
  wires:
  Math Function/1 -> phi/1
  Ro_a/1 -> Product4/2
  Pa/1 -> Product4/1
  Gain2/1 -> Math Function/1
  Product4/1 -> Gain2/1

== system KD_cl_harness_forthao_breach/EGR Valve/SVR EGR/EGR_model/Air Model_map_use/Back-Flow/Cal phi1 ==
  Pm : Inport
  Ro_m : Inport  Port=2
  Gain2 : Gain  Gain=1/(const.Pcab*const.Pcab/const.Rair/const.Tcab)  SaturateOnIntegerOverflow=on  OutDataTypeStr=Inherit: Same as input  ParamDataTypeStr=Inherit: Same as input
  Math Function : Sqrt  Operator=signedSqrt  AlgorithmType=Newton-Raphson  SaturateOnIntegerOverflow=on
  Product4 : Product  Inputs=**  SaturateOnIntegerOverflow=on  RndMeth=Zero  InputSameDT=on  OutDataTypeStr=Inherit: Same as first input
  phi : Outport
  wires:
  Product4/1 -> Gain2/1
  Gain2/1 -> Math Function/1
  Pm/1 -> Product4/1
  Ro_m/1 -> Product4/2
  Math Function/1 -> phi/1

== system KD_cl_harness_forthao_breach/EGR Valve/SVR EGR/EGR_model/Air Model_map_use/Forward-Flow/Cal phi ==
  Pa : Inport
  Ro_a : Inport  Port=2
  Gain2 : Gain  Gain=1/(const.Pcab*const.Pcab/const.Rair/const.Tcab)  SaturateOnIntegerOverflow=on  OutDataTypeStr=Inherit: Same as input  ParamDataTypeStr=Inherit: Same as input
  Math Function : Sqrt  Operator=signedSqrt  AlgorithmType=Newton-Raphson  SaturateOnIntegerOverflow=on
  Product4 : Product  Inputs=**  SaturateOnIntegerOverflow=on  RndMeth=Zero  InputSameDT=on  OutDataTypeStr=Inherit: Same as first input
  phi : Outport
  wires:
  Product4/1 -> Gain2/1
  Gain2/1 -> Math Function/1
  Pa/1 -> Product4/1
  Ro_a/1 -> Product4/2
  Math Function/1 -> phi/1

== system KD_cl_harness_forthao_breach/ctrl_rb_explicit_20131031_v2/expcon/find_region/find_region/leq_check/new_region ==
  rv_in : Inport
  region_in : Inport  Port=2
  Action Port : ActionPort  ActionType=then
  rv_out : Outport
  region_out : Outport  Port=2
  wires:
  rv_in/1 -> rv_out/1
  region_in/1 -> region_out/1

== system KD_cl_harness_forthao_breach/ctrl_rb_explicit_20131031_v2/expcon/find_region/find_region/leq_check/old_region ==
  rv_in : Inport
  region_in : Inport  Port=2
  Action Port : ActionPort  ActionType=else
  rv_out : Outport
  region_out : Outport  Port=2
  wires:
  rv_in/1 -> rv_out/1
  region_in/1 -> region_out/1

== system KD_cl_harness_forthao_breach/ctrl_rb_explicit_20131031_v2/ntestimator/Throttle_Model/Air_Model_map_use/Forward_Flow/Cal_phi ==
  Ro_a : Inport
  Gain2 : Gain  Gain=c_roacorr  SaturateOnIntegerOverflow=on  OutDataTypeStr=Inherit: Same as input  ParamDataTypeStr=Inherit: Same as input
  Saturation : Saturate  UpperLimit=c_inf  LowerLimit=0
      settings: AttributesFormatString=%<LowerLimit>\n%<UpperLimit>
  Sqrt : Sqrt  AlgorithmType=Newton-Raphson  SaturateOnIntegerOverflow=on
  phi : Outport
  wires:
  Sqrt/1 -> phi/1
  Ro_a/1 -> Gain2/1
  Gain2/1 -> Saturation/1
  Saturation/1 -> Sqrt/1

== system KD_cl_harness_forthao_breach/ctrl_rb_explicit_20131031_v2/ntestimator/Throttle_Model/Air_Model_map_use/Forward_Flow/For_Iterator_Subsystem ==
  u : Inport
  sv1 : Inport  Port=2
  sv2 : Inport  Port=3
  arg : Inport  Port=4
  beta : Inport  Port=5
  Demux : Demux  Outputs=2
  Divide : Product  Inputs=*/
  For Iterator : ForIterator  ResetStates=reset  IterationLimit=SVR_EGR_exhat.num_SV
  Gain : Gain  Gain=100
      settings: AttributesFormatString=%<Gain>
  Product{,1..3} (4 alike) : Product  RndMeth=Zero
  Saturation1 : Saturate  UpperLimit=9  LowerLimit=1
      settings: AttributesFormatString=%<LowerLimit>\n%<UpperLimit>
  Selector : Selector  InputPortWidth=SVR_EGR_exhat.num_SV  IndexOptions=Index vector (port)  Indices=[1 3]
  Selector1 : Selector  InputPortWidth=SVR_EGR_exhat.num_SV  IndexOptions=Index vector (port)  Indices=[1 3]
  Selector2 : Selector  InputPortWidth=SVR_EGR_exhat.num_SV  IndexOptions=Index vector (port)  Indices=[1 3]
  Sum : Sum  Inputs=|-+
  Sum1 : Sum  Inputs=+-|
  Sum2 : Sum  Inputs=-|-
  Sum3 : Sum  Inputs=++|
  Unit Delay : UnitDelay  SampleTime=-1
  exp Lookup Table : Lookup  InputValues=SVR_EGR_exhat.exp.x  Table=SVR_EGR_exhat.exp.y  LookUpMeth=Interpolation-Use End Values
      settings: AttributesFormatString=%<LookUpMeth>\n%<InputValues>
  ba : Outport  OutDataTypeStr=single
  wires:
  Saturation1/1 -> [iter]
  For Iterator/1 -> Saturation1/1
  [iter] -> Selector2/2
  [iter] -> Selector1/2
  [iter] -> Selector/2
  Sum3/1 -> ba/1, Unit Delay/1
  Product3/1 -> Sum3/2
  Selector2/1 -> Product3/2
  Gain/1 -> Divide/2
  Product2/1 -> Gain/1
  arg/1 -> Product2/2, Product2/1
  Sum2/1 -> Divide/1
  Product1/1 -> Sum2/2
  Product/1 -> Sum2/1
  Sum1/1 -> Product1/2, Product1/1
  Sum/1 -> Product/2, Product/1
  Demux/2 -> Sum1/1
  Selector1/1 -> Sum1/2
  Demux/1 -> Sum/2
  Selector/1 -> Sum/1
  u/1 -> Demux/1
  beta/1 -> Selector2/1
  sv2/1 -> Selector1/1
  sv1/1 -> Selector/1
  Unit Delay/1 -> Sum3/1
  Divide/1 -> exp Lookup Table/1
  exp Lookup Table/1 -> Product3/1

== matlab function KD_cl_harness_forthao_breach/EGR Valve/SVR EGR/EGR_model/Air Model_map_use/Forward-Flow/SVR_EGR ==
  data: u input; B_A_spd output; num_SV input; Beta input; SV input; arg input
function B_A_spd = fcn(u, num_SV, Beta, SV, arg)
%#eml
Kern=zeros(length(SV),1);
    for n=1:num_SV
        v = SV(n,:).';
        Kern(n)=exp(-(u-v)'*(u-v)/(50*(2*arg^2)));
    end
B_A_spd = Beta.'*Kern;

== matlab function KD_cl_harness_forthao_breach/Turbine/TurbineMap/TurbineMAP1 ==
  data: turb_pres_ratio input; omega_turbo input; p_in_turb input; T_ambient input; T_exh_man input; VNlift input; W_turbine_sim output; Turb_Constants input; TurbFlowCoefs input; TurbTempCoefs input; T_out_turbine output; eta_turb output; A_turbine output; phi output; delta_T_Turbo output; Tq_turbine output
 function [W_turbine_sim, T_out_turbine,eta_turb,A_turbine,phi,delta_T_Turbo,Tq_turbine] = TurbineMap(turb_pres_ratio,omega_turbo,p_in_turb,T_ambient,T_exh_man,VNlift,Turb_Constants, TurbFlowCoefs, TurbTempCoefs)

%% Reference: Turbocharger modelling for Automotive Control Applications by Paul Moraal and Ilya Kolmanovsky
% if T_exh_man <= 0
%     a = 1;
% end
Dia_turb = Turb_Constants(1); %Turbine diameter
Cp = Turb_Constants(2);  % Cp_Air_300K_KJ_per_kg_K
gamma_air = Turb_Constants(3);
eng_Vol = Turb_Constants(4);

PR= turb_pres_ratio;

%% putting saturartions on the blocks
PR = median([0.0001 PR 0.97]); % to avoid Zero-crossing errors

A_turbine  =   TurbFlowCoefs(1) +TurbFlowCoefs(2)*VNlift + TurbFlowCoefs(3)*omega_turbo +TurbFlowCoefs(4)*VNlift.^2 + TurbFlowCoefs(5)*omega_turbo.^2;

p_crit = ((gamma_air + 1)/2)^(gamma_air/(1 -gamma_air));

if PR > p_crit 
    phi_by_At = sqrt(((2*gamma_air)/(gamma_air-1))*(PR^(2/gamma_air) - PR^((gamma_air+1)/gamma_air)));
else
    phi_by_At = 0.6847;  %% check this value
end

phi = phi_by_At * A_turbine ;
phi = median([0.00001 phi 0.2]);
%%
%% to eliminate Zero crossing errors of  simulink
p_in_turb =  median([50 p_in_turb 1000]);
T_exh_man =  median([100 T_exh_man 2000]);

%%
W_turbine_sim = (phi * p_in_turb)/sqrt(T_exh_man); % kgpersec

U_by_C_den = 60*sqrt(2*Cp*T_exh_man*(1- (PR)^((gamma_air-1)/gamma_air)));

U_by_C = (pi* Dia_turb* omega_turbo)/U_by_C_den ;


delta_T_Turbo =  TurbTempCoefs(1) + TurbTempCoefs(2)*U_by_C +TurbTempCoefs(3)*PR...
    + TurbTempCoefs(4)*VNlift +TurbTempCoefs(5)*U_by_C^2 +  TurbTempCoefs(6)*PR^2 +TurbTempCoefs(7)*VNlift^2  ;

% delta_T_Turbo = median([ 0 delta_T_Turbo  250]);
T_out_turbine = T_exh_man - delta_T_Turbo;

eta_turb_num  = 1- (T_out_turbine/T_exh_man);
eta_turb_den = 1 - PR^(0.2857);
eta_turb = eta_turb_num/eta_turb_den ;

% Tq_in Newton meter
% %  Tq in N_m
Tq_turbine = (Cp*W_turbine_sim*delta_T_Turbo*60)/(2*pi*omega_turbo);

== matlab function KD_cl_harness_forthao_breach/Intercooler/Intercooler/MATLAB Function ==
  data: T_in_IC input; T_ambient input; T_out_IC output; ICTempCoefs input
function T_out_IC = InterCoolerMap(T_in_IC,T_ambient,ICTempCoefs)
%#codegen

delT = T_in_IC - T_ambient;
T_out_IC= ICTempCoefs(1)*delT ^2+ ICTempCoefs(2)*delT + ICTempCoefs(3);

== matlab function KD_cl_harness_forthao_breach/Compressor/Comp Map/MATLAB Function ==
  data: pres_Rat input; W_comp output; T_in_comp input; omega_turbo_RPM input; Comp_Constants input; CompPresRatCoefs input; CompEffCoefs input; T_out_comp output; P_comp_W output; pres_Rat1 output; Uc output; Mach output; psi output; k1 output; k2 output; k3 output; PhiC output; Comp_Efficiency output; PhiC1 output; a1 output; a2 output; a3 output; Tq_Compressor output
function [W_comp, T_out_comp,P_comp_W, pres_Rat1,Uc,Mach,psi,k1,k2,k3,PhiC,Comp_Efficiency,PhiC1,a1,a2,a3,Tq_Compressor]   = CompMap(pres_Rat,T_in_comp,omega_turbo_RPM,Comp_Constants,CompPresRatCoefs,CompEffCoefs)

%% Reference: Turbocharger modelling for Automotive Control Applications by Paul Moraal and Ilya Kolmanovsky

dc = Comp_Constants(1); % Compressor Diameter(Outer impeller diameter)
gamma_air = Comp_Constants(2);
R_air = Comp_Constants(3);   % R_specific_air_J_per_kg_kelvin
Cp_Air = Comp_Constants(4);  % Cp_Air_300K_J_per_kg_K
Rho_Air = Comp_Constants(5); % rho_Air_300K_kg_per_m3

x_low = CompPresRatCoefs(1:6);
x_high = CompPresRatCoefs(7:12);

Ntc_cutoff = 25000;
ratio = 0.5*(1 + tanh(((omega_turbo_RPM-Ntc_cutoff)*2*pi)/Ntc_cutoff));
PRcoeffs = (1-ratio)*x_low + ratio*x_high;

% pres_Rat = p_out_comp/p_in_comp;

pres_Rat1 = pres_Rat;
% pres_Rat = median([1 pres_Rat 3]);
% limit pressure ratio accordingly

%% Uc  = Blade speed
Uc = (pi/60)*dc*omega_turbo_RPM;  %% Equation 24

%% Mach = Mach Number
Mach = Uc/(sqrt(gamma_air*R_air*T_in_comp));  %% Equation 26

%% psi = slip factor
psi_num = Cp_Air*T_in_comp*((pres_Rat^((gamma_air -1)/gamma_air))-1);
psi_den = 0.5*Uc*Uc;
psi = psi_num/psi_den;   %% head parameter Equation 23
psi = median([0.0003 psi 10]);

k1 = PRcoeffs(1) + PRcoeffs(2)*Mach;
k2 = PRcoeffs(3) + PRcoeffs(4)*Mach;
k3 = PRcoeffs(5) + PRcoeffs(6)*Mach;

PhiC = ((k3*psi)-k1)/(k2+psi); %%Normalized compressor flow %% Equation 29
PhiC1 = PhiC;
W_comp = PhiC*Rho_Air*(pi/4)*dc*dc*Uc;
W_comp = median([0.0010 W_comp 0.3]);

% % Efficency Calculations

a1 = (CompEffCoefs(1) +  CompEffCoefs(2)*Mach)/(CompEffCoefs(3) - Mach);
a2 = (CompEffCoefs(4) +  CompEffCoefs(5)*Mach)/(CompEffCoefs(6) - Mach);
a3 = (CompEffCoefs(7) +  CompEffCoefs(8)*Mach)/(CompEffCoefs(9) - Mach);

% A = [a1 a2 a3];
Comp_Efficiency = a1*PhiC^2 + a2*PhiC + a3; %%Equation 27
% Comp_Efficiency = median([0.01 Comp_Efficiency 1]);


delta_T_comp = (T_in_comp/Comp_Efficiency)*(pres_Rat^((gamma_air -1)/gamma_air) - 1);
delta_T_comp = median([7  delta_T_comp 150]);

T_out_comp = T_in_comp + delta_T_comp ;  %%Equation 5

P_comp_W = W_comp*Cp_Air*delta_T_comp ; %% power in KW

%% Tq in N-m
Tq_Compressor = (Cp_Air*W_comp*delta_T_comp*60)/(2*pi*omega_turbo_RPM) ;

== matlab function KD_cl_harness_forthao_breach/EGR cooler/EGR Cooler/MATLAB Function ==
  data: T_in_EGR_cooler input; T_out_EGR_cooler output; T_coolant input; W_egr_valve input; EGRbypassflag input; engine_speed_RPM input; EGRCoolerTempCoefs input; EGRCoolerbypassTempCoefs input
function T_out_EGR_cooler   = EGRCoolerMap(T_in_EGR_cooler,T_coolant,W_egr_valve,EGRbypassflag,engine_speed_RPM, EGRCoolerTempCoefs,EGRCoolerbypassTempCoefs )
%#codegen

if EGRbypassflag > 1.5
    
    CoolerPercentEff =  EGRCoolerTempCoefs(1) + EGRCoolerTempCoefs(2)*T_in_EGR_cooler +EGRCoolerTempCoefs(3)*W_egr_valve  +EGRCoolerTempCoefs(4)*engine_speed_RPM...
                    +EGRCoolerTempCoefs(5)*T_in_EGR_cooler^2 + EGRCoolerTempCoefs(6)*W_egr_valve^2 + EGRCoolerTempCoefs(7)*engine_speed_RPM^2;
    
    T_out_EGR_cooler = T_in_EGR_cooler + (T_coolant - T_in_EGR_cooler)*CoolerPercentEff/100;
    
else
    T_out_EGR_cooler = EGRCoolerbypassTempCoefs(1) + EGRCoolerbypassTempCoefs(2)*T_in_EGR_cooler;

end

== matlab function KD_cl_harness_forthao_breach/EGR Throttle/EGR Throttle/Throttle Model2/Air Model_map_use/Back-Flow/SVR_throttle ==
  data: u input; B_A_spd output; num_SV input; Beta input; SV input; arg input
function B_A_spd = fcn(u, num_SV, Beta, SV, arg)
%#eml
Kern=zeros(length(SV),1);
    for n=1:num_SV
        v = SV(n,:).';
        Kern(n)=exp(-(u-v)'*(u-v)/(50*(2*arg^2)));
    end
B_A_spd = Beta.'*Kern;

== matlab function KD_cl_harness_forthao_breach/EGR Valve/SVR EGR/EGR_model/Air Model_map_use/Back-Flow/SVR_EGR ==
  data: u input; B_A_spd output; num_SV input; Beta input; SV input; arg input
function B_A_spd = fcn(u, num_SV, Beta, SV, arg)
%#eml
Kern=zeros(length(SV),1);
    for n=1:num_SV
        v = SV(n,:).';
        Kern(n)=exp(-(u-v)'*(u-v)/(50*(2*arg^2)));
    end
B_A_spd = Beta.'*Kern;

== matlab function KD_cl_harness_forthao_breach/EGR Throttle/EGR Throttle/Throttle Model2/Air Model_map_use/Forward-Flow/SVR_throttle ==
  data: u input; B_A_spd output; num_SV input; Beta input; SV input; arg input
function B_A_spd = fcn(u, num_SV, Beta, SV, arg)
%#eml
Kern=zeros(length(SV),1);
    for n=1:num_SV
        v = SV(n,:).';
        Kern(n)=exp(-(u-v)'*(u-v)/(50*(2*arg^2)));
    end
B_A_spd = Beta.'*Kern;

== matlab function KD_cl_harness_forthao_breach/Combsution/cylinder comp/MATLAB Function ==
  data: W_cyl_out output; omega_engine input; p_in_man input; p_exh_man input; T_in_man input; T_exh_man input; CylConstants input; cylFlowCoefs input; nVol output
function [W_cyl_out,nVol ]= CylinderMap(omega_engine, p_in_man,p_exh_man, T_in_man, T_exh_man,CylConstants,cylFlowCoefs)
%#codegen
% p_in_man
%% check this

%%constraints

T_exh_man =  median([100 T_exh_man 2000]);

cfs = cylFlowCoefs;
nVol = cfs(1) + cfs(2)*omega_engine + cfs(3)*omega_engine^2  + cfs(4)*p_exh_man + cfs(5)*p_in_man + cfs(6)*p_exh_man/sqrt(T_exh_man);   

W_cyl_out = (nVol * p_in_man *omega_engine *CylConstants(1))/(120*CylConstants(2) *T_in_man);

== matlab function KD_cl_harness_forthao_breach/Combsution/Exhaust /MATLAB Function1 ==
  data: omega_engine_rpm input; T_exhaust output; T_in_man input; W_cyl input; u_fuel input; F1_in input; ExhaustTempCoefs input
function T_exhaust    = ExhaustTemp(omega_engine_rpm, T_in_man, W_cyl ,u_fuel, F1_in, ExhaustTempCoefs)
%#codegen

% based on previous engine model fit
% %  no data for doing estimation.
fuelFrac = u_fuel/(W_cyl + u_fuel);
T_exhaust = T_in_man + (ExhaustTempCoefs(1)+ExhaustTempCoefs(2)*fuelFrac +ExhaustTempCoefs(3)*omega_engine_rpm*fuelFrac + ExhaustTempCoefs(4)*F1_in);
